simulink library "RWS_PIDcontroller"  (R2014b)
settings: Solver=ode45  StartTime=0.0  StopTime=10.0  RelTol=1e-3
undefined symbols (not defined in the file or in its folder): ConfParam
libraries: OmegaError x1, Quat2Rot x1, CrossProd x1, Qerror x1
settings Model: Creator=Hp  LastModifiedBy=Hp

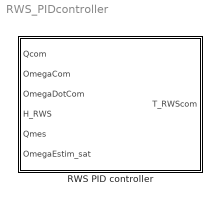
== system RWS_PIDcontroller ==
  RWS PID controller : Subsystem

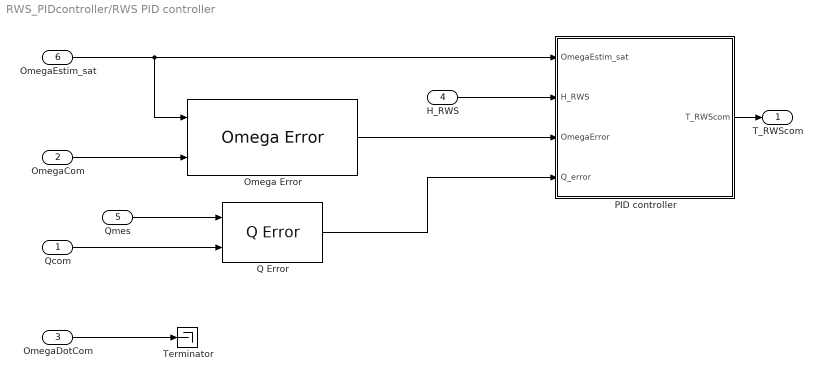
== system RWS_PIDcontroller/RWS PID controller ==
  Qcom : Inport
  OmegaCom : Inport  Port=2
  OmegaDotCom : Inport  Port=3
  H_RWS : Inport  Port=4
  Qmes : Inport  Port=5
  OmegaEstim_sat : Inport  Port=6
  Omega Error : OmegaError/Omega Error
  PID controller : Subsystem
  Q Error : Qerror/Q Error
  Terminator : Terminator
  T_RWScom : Outport
  wires:
  OmegaCom/1 -> Omega Error/2
  OmegaEstim_sat/1 -> PID controller/1(OmegaEstim_sat), Omega Error/1
  Qmes/1 -> Q Error/1
  PID controller/1(T_RWScom) -> T_RWScom/1
  Omega Error/1 -> PID controller/3(OmegaError)
  H_RWS/1 -> PID controller/2(H_RWS)
  Qcom/1 -> Q Error/2
  Q Error/1 -> PID controller/4(Q_error)
  OmegaDotCom/1 -> Terminator/1

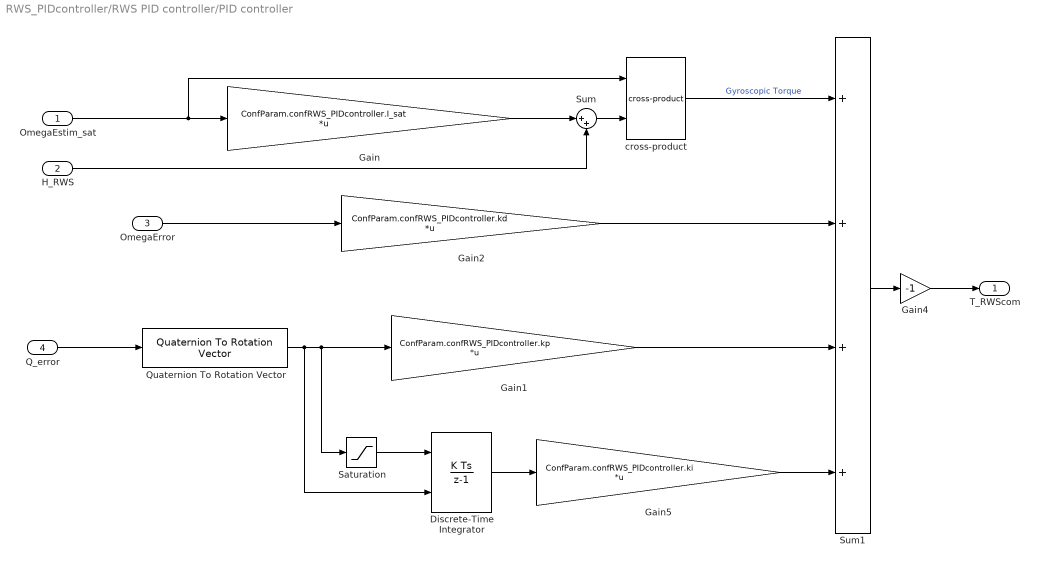
== system RWS_PIDcontroller/RWS PID controller/PID controller ==
  OmegaEstim_sat : Inport
  H_RWS : Inport  Port=2
  OmegaError : Inport  Port=3
  Q_error : Inport  Port=4
  Discrete-Time Integrator : DiscreteIntegrator  InitialConditionSource=external  InitialConditionSetting=State (most efficient)  SampleTime=1/ConfParam.confES.frequency
  Gain : Gain  Gain=ConfParam.confRWS_PIDcontroller.I_sat  Multiplication=Matrix(K*u)
  Gain1 : Gain  Gain=ConfParam.confRWS_PIDcontroller.kp  Multiplication=Matrix(K*u)
  Gain2 : Gain  Gain=ConfParam.confRWS_PIDcontroller.kd  Multiplication=Matrix(K*u)
  Gain4 : Gain  Gain=-1
  Gain5 : Gain  Gain=ConfParam.confRWS_PIDcontroller.ki  Multiplication=Matrix(K*u)
  Quaternion To Rotation Vector : Quat2Rot/Quaternion To Rotation Vector
  Saturation : Saturate  UpperLimit=ConfParam.confRWS_PIDcontroller.ErrorSaturation  LowerLimit=-ConfParam.confRWS_PIDcontroller.ErrorSaturation
  Sum : Sum  Inputs=|++
  Sum1 : Sum  Inputs=++++
  cross-product : CrossProd/cross-product
  T_RWScom : Outport
  wires:
  Gain4/1 -> T_RWScom/1
  Sum1/1 -> Gain4/1
  Gain2/1 -> Sum1/2
  Gain1/1 -> Sum1/3
  Quaternion To Rotation Vector/1 -> Discrete-Time Integrator/2, Saturation/1, Gain1/1
  H_RWS/1 -> Sum/2
  OmegaError/1 -> Gain2/1
  Q_error/1 -> Quaternion To Rotation Vector/1
  Gain/1 -> Sum/1
  cross-product/1 -> Sum1/1  "Gyroscopic Torque"
  OmegaEstim_sat/1 -> Gain/1, cross-product/1
  Sum/1 -> cross-product/2
  Discrete-Time Integrator/1 -> Gain5/1
  Saturation/1 -> Discrete-Time Integrator/1
  Gain5/1 -> Sum1/4
